simulink model "Questao1metodos"  (R2020a)
settings: Solver=VariableStepAuto  StartTime=0.0  StopTime=65  RelTol=1e-3
settings Model: Creator=professor  LastModifiedBy=batis
settings SFSimCC: CustomCodeUndefinedFunction=UseInterfaceOnly

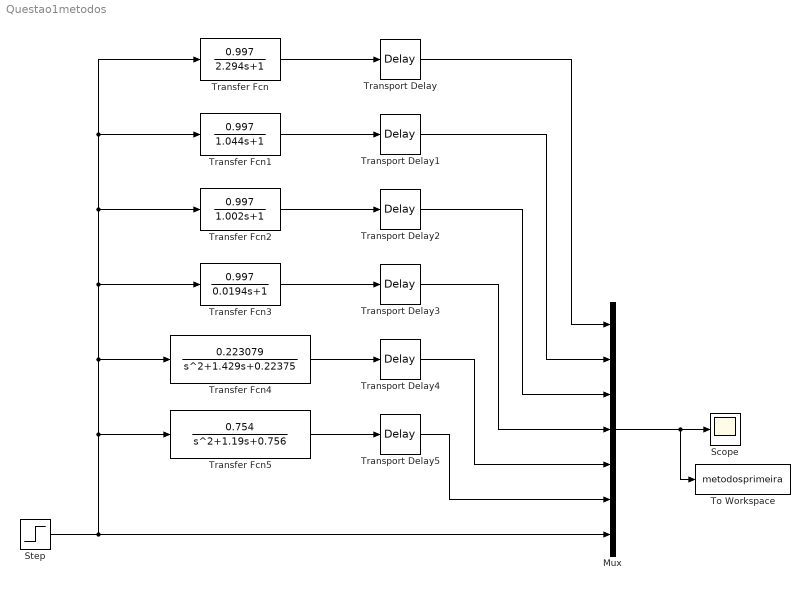
== system Questao1metodos ==
  Mux : Mux  Inputs=7
  Scope : Scope
  Step : Step  Time=11.09  After=3  SampleTime=0
  To Workspace : ToWorkspace  VariableName=metodosprimeira  SaveFormat=Structure With Time  SampleTime=-1
  Transfer Fcn : TransferFcn  Numerator=0.997  Denominator=[2.294 1]
  Transfer Fcn1 : TransferFcn  Numerator=0.997  Denominator=[1.044 1]
  Transfer Fcn2 : TransferFcn  Numerator=0.997  Denominator=[1.002 1]
  Transfer Fcn3 : TransferFcn  Numerator=0.997  Denominator=[0.0194 1]
  Transfer Fcn4 : TransferFcn  Numerator=0.223079  Denominator=[1 1.429 0.22375]
  Transfer Fcn5 : TransferFcn  Numerator=0.754  Denominator=[1 1.19 0.756]
  Transport Delay : TransportDelay  DelayTime=0.06
  Transport Delay1 : TransportDelay  DelayTime=0.846
  Transport Delay2 : TransportDelay  DelayTime=0.6317
  Transport Delay3 : TransportDelay  DelayTime=0.002016
  Transport Delay4 : TransportDelay  DelayTime=18.05
  Transport Delay5 : TransportDelay  DelayTime=10.52
  wires:
  Transport Delay2/1 -> Mux/3
  Transport Delay5/1 -> Mux/6
  Transport Delay4/1 -> Mux/5
  Transport Delay1/1 -> Mux/2
  Transport Delay/1 -> Mux/1
  Transport Delay3/1 -> Mux/4
  Transfer Fcn4/1 -> Transport Delay4/1
  Transfer Fcn/1 -> Transport Delay/1
  Transfer Fcn5/1 -> Transport Delay5/1
  Transfer Fcn1/1 -> Transport Delay1/1
  Transfer Fcn2/1 -> Transport Delay2/1
  Mux/1 -> To Workspace/1, Scope/1
  Step/1 -> Transfer Fcn/1, Transfer Fcn1/1, Transfer Fcn2/1, Transfer Fcn3/1, Transfer Fcn4/1, Transfer Fcn5/1, Mux/7
  Transfer Fcn3/1 -> Transport Delay3/1
